simulink model "sm_worm_gear_assembly_testrig"  (R2026a)
settings: Solver=VariableStepAuto  MaxStep=1e-2  EnableMultiTasking=on
undefined symbols (not defined in the file or in its folder): Hand, Right
libraries: sm_lib x3, nesl_utility x2, Multibody_Parts_Lib x1
CloseFcn:
  | try,close(h1_sm_worm_gear_assembly_testrig),end
  | clear h1_sm_worm_gear_assembly_testrig
  | 
  | clear simlog_sm_worm_gear_assembly_testrig
  | clear logsout_sm_worm_gear_assembly_testrig
Description:
  | Worm Gear Assembly Testrig
  | 
  | Copyright 2017-2026 The MathWorks, Inc.
settings Model: Creator=smiller  LastModifiedBy=smiller
settings DataIOCC: SignalLoggingName=logsout_sm_worm_gear_assembly_testrig
settings DebuggingCC: PregeneratedLibrarySubsystemCodeDiagnostic=none
settings SimscapeCC: SimscapeNormalizeSystem=off  SimscapeNominalValues="[{\"value\":\"1\",\"unit\":\"A\"},{\"value\":\"1\",\"unit\":\"bar\"},{\"value\":\"1\",\"unit\":\"cm^2\"},{\"value\":\"1\",\"unit\":\"cm^3/s\"},{\"value\":\"1\",\"unit\":\"kJ/kg\"},{\"value\":\"1\",\"unit\":\"kW\"},{\"value\":\"1\",\"unit\":\"l\"},{\"value\":\"1\",\"unit\":\"N\"},{\"value\":\"1\",\"unit\":\"N*m\"},{\"value\":\"1\",\"unit\":\"V\"}]"  SimscapeLogSimulationStatistics=on  SimscapeLogName=simlog_sm_worm_gear_assembly_testrig
settings ConfigurationSet: Description=SimMechanics 2G
settings DiagnosticsConfigSet: SimMechanicsUnconnectedFramePorts=none
settings ExplorerConfigSet: InternalSimMechanicsExplorerSettings="<ExplorerConfiguration><canonicalview>planar_xy</canonicalview><AnimationSetting><BasePlaybackSpeed>1.0</BasePlaybackSpeed><PlaybackSpeedFactor>1.0</PlaybackSpeedFactor></AnimationSetting><TilePanel><TileInfo><Tiles Columns=\"1\" Count=\"1\" Rows=\"1\"><Column Left=\"2\" Weight=\"1\"/><Column Left=\"470\"/><Row Top=\"2\" Weight=\"1\"/><Row Top=\"477\"/><Tile Height=\"1\" Width=\"1\" X=\"0\" Y=\"0\"/></Tiles></TileInfo><SceneInfo><SceneViewer><BGColor><R>1</R><G>1</G><B>1</B></BGColor><Camera><DoPerspective>off</DoPerspective><Position><X>-0.73056719793560465</X><Y>0.17365895503578019</Y><Z>0.662790382531667</Z></Position><Center><X>0.0020893235873772889</X><Y>0.036303358738908165</Y><Z>-0.0038038430927192718</Z></Center><Up><X>0.07560646522266555</X><Y>0.98978708011987249</Y><Z>-0.12085196913708666</Z></Up><ViewLimDist>1</ViewLimDist><YLim>0.052264586500823502</YLim><XLim>0.05147949614566092</XLim></Camera></SceneViewer></SceneInfo></TilePanel><MechEditorPanel><Cameras/><GfxPanelCameraMap/><VideoCreator><PlaybackSpeedRatio>1.0</PlaybackSpeedRatio><FrameRate>30</FrameRate><VideoFormat>Motion JPEG AVI</VideoFormat><FrameSize>auto</FrameSize></VideoCreator></MechEditorPanel></ExplorerConfiguration>"

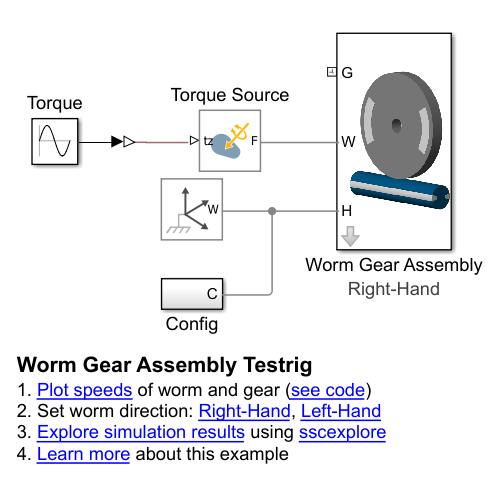
[thumbnail: Simulink's stored preview of the top-level diagram]
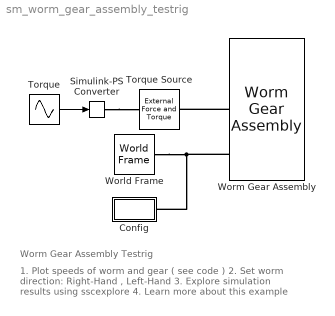
== system sm_worm_gear_assembly_testrig ==
  note: Worm Gear Assembly Testrig
  note: 1. Plot speeds of worm and gear ( see code )
      | 2. Set worm direction: Right-Hand , Left-Hand
      | 3. Explore simulation results using sscexplore
      | 4. Learn more about this example
  Config : Subsystem
  Simulink-PS Converter : nesl_utility/Simulink-PS Converter  PhysicalDomain=network_engine_domain  SubClassName=ps_input  LeftPortType=input  RightPortType=output  PseudoPeriodic=off  Frequencies=[]  NoiseDistribution=none  NoiseParameters=[]  Unit=1  AffineConversion=off  FilteringAndDerivatives=zero  SimscapeFilterOrder=1  InputFilterTimeConstant=0.001  UdotUserProvided=1
  Torque : Sin  Amplitude=10  Frequency=pi/2  Phase=pi/2  SampleTime=0
  Torque Source : sm_lib/Forces and Torques/External Force and Torque  EnableForceX=off  EnableForceY=off  EnableForceZ=off  EnableForce=off  ForceResolutionFrame=AttachedFrame  EnableTorqueX=off  EnableTorqueY=off  EnableTorqueZ=on  EnableTorque=off  TorqueResolutionFrame=AttachedFrame
  World Frame : sm_lib/Frames and Transforms/World Frame
  Worm Gear Assembly : Multibody_Parts_Lib/Gears/Assemblies/Worm Gear Assembly  Tag=PublishSubsystem  popup_worm_dir_asy=Right-Hand  worm_lead_angle_asy=4.2  gear_ra_asy=37.5e-3  gear_th_asy=9e-3  gear_hr_asy=5e-3  gear_rho_asy=7000  gear_clr_asy=[0.6 0.6 0.6]  gear_opc_asy=1  gear_visc_frict_asy=1e-2  g_popup_markings=Two  g_mark_radius_range=[0.7 0.9]  g_mark_angle_range=60  g_mark_color=[1 1 1]  worm_rad_asy=8.5e-3  worm_len_asy=85e-3  worm_rho_asy=7000  worm_color_asy=[0.0 0.4 0.6]  worm_opc_asy=1  worm_visc_frict_asy=1e-2  w_popup_markings=Two  w_mark_radius_range=[0.5 1.01]  w_mark_length_range=1.005  w_mark_angle_range=30  w_mark_color=[1 1 1]
      settings: AttributesFormatString=%<popup_worm_dir_asy>  SourceProductName=Simscape Multibody Parts Library
  wires:
  Torque/1 -> Simulink-PS Converter/1
  connections:
  World Frame/RConn1 -- Worm Gear Assembly/LConn3 -- Config/RConn1
  Worm Gear Assembly/LConn2 -- Torque Source/RConn1
  Simulink-PS Converter/RConn1 -- Torque Source/LConn1

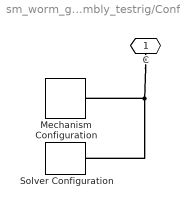
== system sm_worm_gear_assembly_testrig/Config ==
  Mechanism Configuration : sm_lib/Utilities/Mechanism Configuration  UniformGravity=Constant  GravityVector=[0 0 -9.80665]  GravityVectorUnits=m/s^2  LinearizationDelta=0.001  JointModeTransitionNonlinearIterations=2
  Solver Configuration : nesl_utility/Solver Configuration  PhysicalDomain=network_engine_domain  SubClassName=solver  LeftPortType=input  RightPortType=generic  Tones=[]  Harmonics=[]  SimulateNoise=off  Profile=off  UseLocalSampling=off  EnableSwitchedLinearOptims=on  FrequencyDomain=off  UseCCode=off  RelTol=0.001  AbsTol=1e-06  MinStep=1e-09  ToWorkspace=off  RevertToSquareIcSolve=off  NumHomotopyIterations=100  PhasorMode=off  PhasorModeNumHarmonics=1  ConsistencySolver=NEWTON_FTOL  CanonicalOrdering=UNORDERED  OptimizeIntermediates=UNOPTIMIZED  IndexReductionMethod=DerivativeReplacement  DoDC=off  ResidualTolerance=1e-09  ConsistencyTolSource=GLOBAL  ConsistencyAbsTol=0.001  ConsistencyRelTol=0.001  ConsistencyTolFactor=0.001  UseLocalSolver=off  LocalSolverChoice=NE_BACKWARD_EULER_ADVANCER  ResolveIndetEquations=on  FunctionEvalNumThread=1  LocalSolverSampleTime=0.001  DoFixedCost=off  MaxNonlinIter=3  MaxModeIter=2  ComputeImpulses=off  ImpulseIterations=2  LinearAlgebra=Sparse  LinearAlgebraNumThread=0  EquationFormulation=NE_TIME_EF  DelaysMemoryBudget=1024  AutomaticFiltering=on  FilteringTimeConstant=0.001  PartitionStorageMethod=AS_NEEDED  PartitionMemoryBudget=1024  PartitionMethod=FAST  MultibodyUseLocalSolver=off  MultibodyLocalSolverChoice=ODE1  MultibodyLocalSolverSampleTime=0.001
  C : PMIOPort  Side=Right
  connections:
  Solver Configuration/RConn1 -- C/RConn1 -- Mechanism Configuration/RConn1
